simulink library "mblibv1"  (Simulink 6.0)
settings: Solver=ode45  StartTime=0.0  StopTime=10.0  RelTol=1e-3
undefined symbols (not defined in the file or in its folder): gcbh, mech_support
libraries: mblibv1 x10, simulink x5
(part 2 of 2)

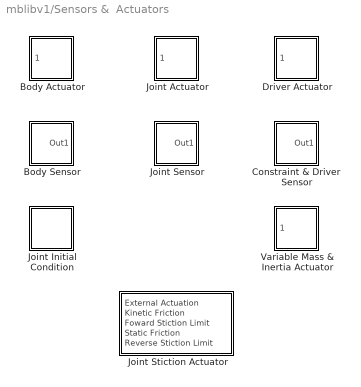
== system mblibv1/Sensors &  Actuators ==
  Body Actuator : Subsystem  LoadFcn=mech_support('LoadFcn',gcbh);  StartFcn=mech_support('StartFcn',gcbh);  StopFcn=mech_support('StopFcn',gcbh);  Opaque=on  mask(msb){PhysicalDomain=Mechanical, PortType=blob, ActuationStyle=Force, AngleUnits=deg, ArcVelocityUnits=deg/s, ArcAccelerationUnits=deg/s^2, CoordPositionUnits=m, VelocityUnits=m/s, AccelerationUnits=m/s^2, ForceUnits=N, TorqueUnits=N-m, ActiveIO=off, Width=1, ClassName=BodyActuatorForceTorque, DialogClass=MechanicalActuatorBlock, ReferenceFrame=Absolute (INERTIAL), Angle=off, CoordPosition=on, Force=on, Torque=off}
      mask help: Actuates a Body with generalized force/torque signal. Vector components specified with respect to reference coordinate system. Input is a Simulink signal. For Body motion or initial condition actuation, press Help.
      mask init:
      | mech_initIO(gcbh);
      settings: CopyFcn=mech_support('CopyFcn',gcbh);  DeleteFcn=mech_support('deleteFcn',gcbh);  UndoDeleteFcn=mech_support('undoDeleteFcn',gcbh);  ModelCloseFcn=mech_support('modelCloseFcn',gcbh);  NameChangeFcn=mech_support('nameChangeFcn',gcbh);  OpenFcn=mech_support('openFcn',gcbh);  CloseFcn=mech_support('CloseFcn',gcbh);
      mask Help: web(mech_help('bodyactuator'))
      mask Display: image(mech_getIcon('b_act.bmp', 'Mechanical'),'center');
  Body Sensor : Subsystem  LoadFcn=mech_support('LoadFcn',gcbh);  StartFcn=mech_support('StartFcn',gcbh);  StopFcn=mech_support('StopFcn',gcbh);  Opaque=on  mask(msb){PhysicalDomain=Mechanical, PortType=blob, Muxed=on, Pose=off, Angle=on, AngleUnits=deg, ArcVelocity=off, ArcVelocityUnits=deg/s, ArcAcceleration=off, ArcAccelerationUnits=deg/s^2, CoordPosition=on, CoordPositionUnits=m, Velocity=off, VelocityUnits=m/s, Acceleration=off, AccelerationUnits=m/s^2, Quaternion=on, QuaternionDT=off, QuaternionDDT=off, QuaternionUnits=off, OutputVector=[1], ActiveIO=off, Width=1, ClassName=BodySensor, DialogClass=MechanicalSensorBlock, ReferenceFrame=Absolute (INERTIAL)}
      mask help: Measures linear/angular position, velocity, and/or acceleration of a Body with respect to a specified coordinate system. Optional rotation matrix for Body orientation. Output is Simulink signal. Multiple output signals can be bundled into one signal.
      mask init:
      | mech_initIO(gcbh);mech_construct(gcbh);
      settings: CopyFcn=mech_support('CopyFcn',gcbh);  DeleteFcn=mech_support('deleteFcn',gcbh);  UndoDeleteFcn=mech_support('undoDeleteFcn',gcbh);  ModelCloseFcn=mech_support('modelCloseFcn',gcbh);  NameChangeFcn=mech_support('nameChangeFcn',gcbh);  OpenFcn=mech_support('openFcn',gcbh);  CloseFcn=mech_support('CloseFcn',gcbh);
      mask Help: web(mech_help('bodysensor'))
      mask Display: image(mech_getIcon('b_sensor.bmp', 'Mechanical'),'center');
  Constraint & Driver  Sensor : Subsystem  LoadFcn=mech_support('LoadFcn',gcbh);  StartFcn=mech_support('StartFcn',gcbh);  StopFcn=mech_support('StopFcn',gcbh);  Opaque=on  mask(msb){PhysicalDomain=Mechanical, ClassName=ConstraintSensor, DialogClass=ConstraintSensorBlock, SensedSide=Base, ReferenceFrame=Absolute (World), ReactionForce=on, ForceUnits=N, ReactionMoment=on, MomentUnits=N-m, Muxed=on, OutputVector=[3 3], ActiveIO=off, Width=1}
      mask help: Measures Constraint/Driver reaction forces/torques between the base (B) and follower (F) Bodies with respect to the selected coordinate system. Outputs are Simulink signals. Force and torque vectors can be bundled into one signal.
      mask init:
      | mech_initIO(gcbh);mech_construct(gcbh);
      settings: CopyFcn=mech_support('CopyFcn',gcbh);  DeleteFcn=mech_support('deleteFcn',gcbh);  UndoDeleteFcn=mech_support('undoDeleteFcn',gcbh);  ModelCloseFcn=mech_support('modelCloseFcn',gcbh);  NameChangeFcn=mech_support('nameChangeFcn',gcbh);  OpenFcn=mech_support('openFcn',gcbh);  CloseFcn=mech_support('CloseFcn',gcbh);
      mask Help: web(mech_help('constraintdriversensor'))
      mask Display: image(mech_getIcon('constr_sen.bmp', 'Mechanical'),'center');
  Driver Actuator : Subsystem  LoadFcn=mech_support('LoadFcn',gcbh);  StartFcn=mech_support('StartFcn',gcbh);  StopFcn=mech_support('StopFcn',gcbh);  Opaque=on  mask(msb){PhysicalDomain=Mechanical, ClassName=ConstraintActuator, DialogClass=ConstraintActuatorBlock, PortType=blob, AngleUnits=deg, ArcVelocityUnits=deg/s, ArcAccelerationUnits=deg/s^2, CoordPositionUnits=m, VelocityUnits=m/s, AccelerationUnits=m/s^2, ActiveIO=off, Width=1}
      mask help: Inputs position, velocity, and acceleration Simulink signals to Driver to drive relative motion between the base (B) and follower (F) Bodies. Base-follower sequence and joint axis determine sign of forward motion. Input signals must be bundled into one signal.
      mask init:
      | mech_initIO(gcbh);
      settings: CopyFcn=mech_support('CopyFcn',gcbh);  DeleteFcn=mech_support('deleteFcn',gcbh);  UndoDeleteFcn=mech_support('undoDeleteFcn',gcbh);  ModelCloseFcn=mech_support('modelCloseFcn',gcbh);  NameChangeFcn=mech_support('nameChangeFcn',gcbh);  OpenFcn=mech_support('openFcn',gcbh);  CloseFcn=mech_support('CloseFcn',gcbh);
      mask Help: web(mech_help('driveractuator'))
      mask Display: image(mech_getIcon('driv_act.bmp', 'Mechanical'),'center');
  Joint Actuator : Subsystem  LoadFcn=mech_support('LoadFcn',gcbh);  StartFcn=mech_support('StartFcn',gcbh);  StopFcn=mech_support('StopFcn',gcbh);  Opaque=on  mask(msb){PhysicalDomain=Mechanical, PortType=blob, ActuationStyle=Force, AngleUnits=deg, ArcVelocityUnits=deg/s, ArcAccelerationUnits=deg/s^2, CoordPositionUnits=m, VelocityUnits=m/s, AccelerationUnits=m/s^2, ForceUnits=N, TorqueUnits=N-m, ActiveIO=off, Width=1, ClassName=JointActuator, DialogClass=MechanicalActuatorBlock, Primitive=None, ReferenceFrame=Absolute (INERTIAL)}
      mask help: Actuates a Joint primitive with generalized force/torque or linear/angular position, velocity, and acceleration motion signals. Base-follower sequence and joint axis determines sign of forward motion. Inputs are Simulink signals. Motion input signals must be bundled into one signal. Connect to Joint block to see Connected to primitive list.
      mask init:
      | mech_initIO(gcbh);
      settings: CopyFcn=mech_support('CopyFcn',gcbh);  DeleteFcn=mech_support('deleteFcn',gcbh);  UndoDeleteFcn=mech_support('undoDeleteFcn',gcbh);  ModelCloseFcn=mech_support('modelCloseFcn',gcbh);  NameChangeFcn=mech_support('nameChangeFcn',gcbh);  OpenFcn=mech_support('openFcn',gcbh);  CloseFcn=mech_support('CloseFcn',gcbh);
      mask Help: web(mech_help('jointactuator'))
      mask Display: image(mech_getIcon('j_act.bmp', 'Mechanical'),'center');
  Joint Initial Condition : Subsystem  LoadFcn=mech_support('LoadFcn',gcbh);  StartFcn=mech_support('StartFcn',gcbh);  StopFcn=mech_support('StopFcn',gcbh);  Opaque=on  mask(msb){PhysicalDomain=Mechanical, ClassName=InitialCondition, DialogClass=InitialConditionBlock, Primitive=, CoordPosition=, Velocity=, AngleUnits=, ArcVelocityUnits=, CoordPositionUnits=, VelocityUnits=, InitialConditions=P1$false$0$m$rad$0$m/s$rad/s#P2$false$0$m$rad$0$m/s$rad/s#P3$false$0$m$rad$0$m/s$rad/s#R1$false$0$m$rad$0$m/s$rad/s#R2$false$0$m$rad$0$m/s$rad/s#R3$false$0$m$rad$0$m/s$rad/s#S$false$0$m$rad$0$m/s$rad/s}
      mask help: Sets the initial linear/angular position and velocity of some or all of the primitives in a Joint. Connect to a Joint to see a list of its primitives.
      settings: CopyFcn=mech_support('CopyFcn',gcbh);  DeleteFcn=mech_support('deleteFcn',gcbh);  UndoDeleteFcn=mech_support('undoDeleteFcn',gcbh);  ModelCloseFcn=mech_support('modelCloseFcn',gcbh);  PreSaveFcn=mech_support('PreSaveFcn');  PostSaveFcn=mech_support('PostSaveFcn');  NameChangeFcn=mech_support('nameChangeFcn',gcbh);  OpenFcn=mech_support('openFcn',gcbh);  CloseFcn=mech_support('CloseFcn',gcbh);
      mask Help: web(mech_help('jointinitialconditionactuator'))
      mask Display: image(mech_getIcon('init_cond.bmp', 'Mechanical'),'center');
  Joint Sensor : Subsystem  LoadFcn=mech_support('LoadFcn',gcbh);  StartFcn=mech_support('StartFcn',gcbh);  StopFcn=mech_support('StopFcn',gcbh);  Opaque=on  mask(msb){PhysicalDomain=Mechanical, PortType=blob, Muxed=on, Pose=off, Angle=on, AngleUnits=deg, ArcVelocity=off, ArcVelocityUnits=deg/s, ArcAcceleration=off, ArcAccelerationUnits=deg/s^2, CoordPosition=on, CoordPositionUnits=m, Velocity=off, VelocityUnits=m/s, Acceleration=off, AccelerationUnits=m/s^2, Quaternion=on, QuaternionDT=off, QuaternionDDT=off, QuaternionUnits=off, OutputVector=[1], ActiveIO=off, Width=1, ClassName=JointSensor, DialogClass=MechanicalSensorBlock, Primitive=None, Force=off, ForceUnits=N, Torque=off, TorqueUnits=N-m, ReferenceFrame=Absolute (INERTIAL), ReactionSensedSide=Base, ReactionReferenceFrame=Absolute (World), ReactionForce=off, ReactionForceUnits=N, ReactionMoment=off, ReactionMomentUnits=N-m}
      mask help: Measures linear/angular position, velocity, acceleration, computed force/torque and/or reaction force/torque of a Joint primitive. Spherical measured by quaternion. Base-follower sequence and joint axis determine sign of forward motion. Outputs are Simulink signals. Multiple output signals can be bundled into one signal. Connect to Joint block to see Connected to primitive list.
      mask init:
      | mech_initIO(gcbh);mech_construct(gcbh);
      settings: CopyFcn=mech_support('CopyFcn',gcbh);  DeleteFcn=mech_support('deleteFcn',gcbh);  UndoDeleteFcn=mech_support('undoDeleteFcn',gcbh);  ModelCloseFcn=mech_support('modelCloseFcn',gcbh);  NameChangeFcn=mech_support('nameChangeFcn',gcbh);  OpenFcn=mech_support('openFcn',gcbh);  CloseFcn=mech_support('CloseFcn',gcbh);
      mask Help: web(mech_help('jointsensor'))
      mask Display: image(mech_getIcon('j_sensor.bmp', 'Mechanical'),'center');
  Joint Stiction Actuator : Subsystem  LoadFcn=mech_support('LoadFcn',gcbh);  StartFcn=mech_support('StartFcn',gcbh);  StopFcn=mech_support('StopFcn',gcbh);  Opaque=on  mask(msb){PhysicalDomain=Mechanical, PortType=blob, ActuationStyle=Force, AngleUnits=deg, ArcVelocityUnits=deg/s, ArcAccelerationUnits=deg/s^2, CoordPositionUnits=m, VelocityUnits=m/s, AccelerationUnits=m/s^2, ForceUnits=N, TorqueUnits=N-m, ActiveIO=off, Width=1, ClassName=JointStictionActuator, DialogClass=EventActuatorBlock, Primitive=None, FrictionalForceUnits=N, ExternalForceUnits=N, FrictionalTorqueUnits=N-m, ExternalTorqueUnits=N-m, LockingTolerance=1e-2}
      mask help: Actuates a Joint primitive with stiction force/torque. Locked if static friction remains within range of forward and reverse stiction limits. External actuation and kinetic friction require units. Velocity threshold in MKS (SI) units. Base-follower sequence and joint axis determine sign of forward motion. Inputs are Simulink signals. Connect to Joint block to see the Connected to primitive list.
      mask init:
      | mech_initIO(gcbh);
      settings: CopyFcn=mech_support('CopyFcn',gcbh);  DeleteFcn=mech_support('deleteFcn',gcbh);  UndoDeleteFcn=mech_support('undoDeleteFcn',gcbh);  ModelCloseFcn=mech_support('modelCloseFcn',gcbh);  NameChangeFcn=mech_support('nameChangeFcn',gcbh);  OpenFcn=mech_support('openFcn',gcbh);  CloseFcn=mech_support('CloseFcn',gcbh);
      mask Help: web(mech_help('jointstictionactuator'))
  Variable Mass & Inertia Actuator : Subsystem  LoadFcn=mech_support('LoadFcn',gcbh);  StartFcn=mech_support('StartFcn',gcbh);  StopFcn=mech_support('StopFcn',gcbh);  Opaque=on  mask(msb){PhysicalDomain=Mechanical, PortType=blob, ActuationStyle=MassInertia, AngleUnits=deg, ArcVelocityUnits=deg/s, ArcAccelerationUnits=deg/s^2, CoordPositionUnits=m, VelocityUnits=m/s, AccelerationUnits=m/s^2, ForceUnits=N, TorqueUnits=N-m, ActiveIO=off, Width=1, ClassName=BodyActuatorMassInertia, DialogClass=VariableMassInertiaActuatorBlock, Mass=on, Inertia=off, ReferenceFrame=Local (body CS), MassUnits=kg, InertiaUnits=kg*m^2}
      mask help: Varies the mass and/or inertia tensor of the connected Body. Attaches to the connected Body coordinate system (CS) an invisible body of time-varying mass and/or inertia tensor. Time-varying mass and inertia tensor are transformed from the attached CS to the new common center of gravity and added to the values supplied in the Body dialog. Multiple time-varying masses and inertia tensors can be added to a Body. Input is a Simulink signal with one, nine, or ten components.
      mask init:
      | mech_initIO(gcbh);
      settings: CopyFcn=mech_support('CopyFcn',gcbh);  DeleteFcn=mech_support('deleteFcn',gcbh);  UndoDeleteFcn=mech_support('undoDeleteFcn',gcbh);  ModelCloseFcn=mech_support('modelCloseFcn',gcbh);  NameChangeFcn=mech_support('nameChangeFcn',gcbh);  OpenFcn=mech_support('openFcn',gcbh);  CloseFcn=mech_support('CloseFcn',gcbh);
      mask Help: web(mech_help('variablemassinertiaactuator'))
      mask Display: image(mech_getIcon('vmi_act.bmp', 'Mechanical'),'center');

== system mblibv1/Utilities ==
  Continuous Angle : Subsystem  Tag=Factory continuousAngle  AncestorBlock=plantlib/Smooth Angle  mask{rad=deg, rads=deg/s}
      mask prompts: rad "Angle measured in:"; rads "Rate measured in:"
      mask help: Outputs a continuous, unbounded angle given a discontinuous, bounded angle and the angular velocity. Choose units for the angle and the angular velocity (rate).
      mask Help: web(mech_help('continuousangle'))
      mask StyleString: popup(rad|deg),popup(rad/s|deg/s)
  Convert from Rotation Matrix to Virtual Reality Toolbox : S-Function  Tag=Pose2VR  FunctionName=sfun_pose2vr
      mask Type: RotationMatrix2VR
      mask Description: Transforms body orientation representations. Converts a 3 x 3 rotation matrix to a 4-component vector, a spatial unit vector plus a rotation angle about that vector. The input must be a 9-element vector representing the rotation matrix column-wise. The output format is that required by the Virtual Reality Toolbox for specifying orientation.
      mask Help: web(mech_help('rotationmatrix2vr'))
      mask Display: disp('RotationMatrix2VR')
  Mechanical Branching Bar : PMComponent  LoadFcn=mech_support('LoadFcn',gcbh);  StartFcn=mech_support('StartFcn',gcbh);  StopFcn=mech_support('StopFcn',gcbh);  PhysicalDomain=mechanical  SubClassName=Unknown  LeftPortType=blob  RightPortType=blob  LConnTagsString=_newl0  RConnTagsString=SA0|SA1  mask(msb){ClassName=BranchingBar, DialogClass=MechanicalBranchingBarBlock, NumSAPorts=2}
      mask help: Maps multiple sensor/actuator lines to one sensor/actuator port. On a Body, connects many sensor/actuator lines to one Body coordinate system. On a Joint, Constraint, or Driver, connects many sensor/actuator lines to one sensor/actuator port. Allows choice of primitives on Joints, reactions forces/torques on Constraints and Drivers, and motion actuation on Drivers.
      settings: CopyFcn=mech_support('CopyFcn',gcbh);  DeleteFcn=mech_support('deleteFcn',gcbh);  UndoDeleteFcn=mech_support('undoDeleteFcn',gcbh);  ModelCloseFcn=mech_support('modelCloseFcn',gcbh);  NameChangeFcn=mech_support('nameChangeFcn',gcbh);  OpenFcn=mech_support('openFcn',gcbh);  CloseFcn=mech_support('CloseFcn',gcbh);
      mask Help: web(mech_help('mechanicalbranchingbar'))
      mask Display: image(mech_getIcon('branchingbar.bmp', 'Mechanical'));
  Connection Port : PMIOPort  Tag=PMCPort  Port=1  Side=Left

== system mblibv1/Bodies/Ground ==
  out : PMIOPort  Port=1  Side=Right

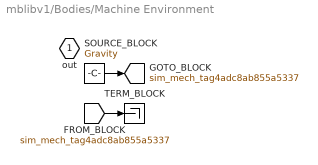
== system mblibv1/Bodies/Machine Environment ==
  SOURCE_BLOCK : Constant  Value=Gravity
  TERM_BLOCK : Terminator
  out : PMIOPort  Port=1  Side=Right
  tag scope: sim_mech_tag4adc8ab855a5337=global
  wires:
  SOURCE_BLOCK/1 -> [sim_mech_tag4adc8ab855a5337]
  [sim_mech_tag4adc8ab855a5337] -> TERM_BLOCK/1

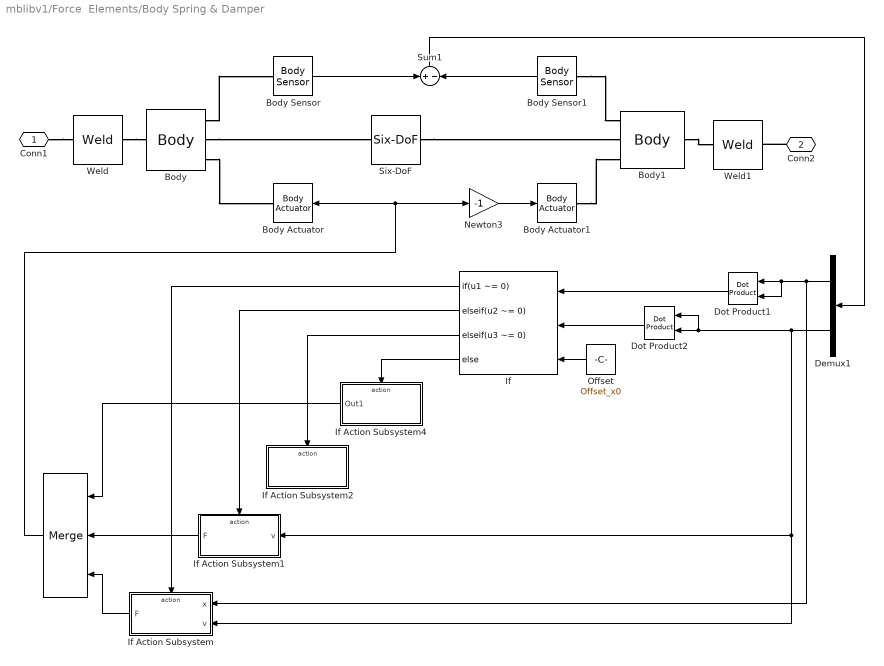
== system mblibv1/Force  Elements/Body Spring & Damper ==
  " " : Merge  Orientation=left  Inputs=3
  Body : mblibv1/Bodies/Body  PhysicalDomain=mechanical  SubClassName=Unknown  LeftPortType=workingframe  RightPortType=workingframe  LConnTagsString=CS1  RConnTagsString=CS2|CS3|CS4  DialogClass=MechanicalBodyBlock  Mass=0  MassUnits=kg  InertiaUnits=kg*m^2  Inertia=zeros(3, 3)  Shape=Cylinder  ShapeDims=[1 1]  ShapeUnits=m  ShapeUse=false  Density=1  DensityUnits=kg/m^3  DensityUse=false  CG=Left$CG$[0 0 0]$CS1$CS1$m$[0 0 0]$Euler X-Y-Z$deg$WORLD$false  WorkingFrames=Left$CS1$[0 0 0]$ADJOINING$ADJOINING$m$[0 0 0]$Euler X-Y-Z$deg$WORLD$true#Right$CS2$[0 0 0]$CS1$CS1$m$[0 0 0]$Euler X-Y-Z$deg$WORLD$true#Right$CS3$[0 0 0]$CS1$CS1$m$[0 0 0]$Euler X-Y-Z$deg$WORLD$true#Right$CS4$[0 0 0]$CS1$CS1$m$[0 0 0]$Euler X-Y-Z$deg$WORLD$true
  Body Actuator : mblibv1/Sensors &  Actuators/Body Actuator  Orientation=left  Opaque=on  PhysicalDomain=Mechanical  PortType=blob  ActuationStyle=Force  AngleUnits=deg  ArcVelocityUnits=deg/s  ArcAccelerationUnits=deg/s^2  CoordPositionUnits=m  VelocityUnits=m/s  AccelerationUnits=m/s^2  ForceUnits=N  TorqueUnits=N-m  ActiveIO=off  Width=3  DialogClass=MechanicalActuatorBlock  ReferenceFrame=Absolute (INERTIAL)  Angle=off  CoordPosition=on  Force=on  Torque=off
  Body Actuator1 : mblibv1/Sensors &  Actuators/Body Actuator  Opaque=on  PhysicalDomain=Mechanical  PortType=blob  ActuationStyle=Force  AngleUnits=deg  ArcVelocityUnits=deg/s  ArcAccelerationUnits=deg/s^2  CoordPositionUnits=m  VelocityUnits=m/s  AccelerationUnits=m/s^2  ForceUnits=N  TorqueUnits=N-m  ActiveIO=off  Width=3  DialogClass=MechanicalActuatorBlock  ReferenceFrame=Absolute (INERTIAL)  Angle=off  CoordPosition=on  Force=on  Torque=off
  Body Sensor : mblibv1/Sensors &  Actuators/Body Sensor  Opaque=on  PhysicalDomain=Mechanical  PortType=blob  Muxed=on  Pose=off  Angle=on  AngleUnits=deg  ArcVelocity=off  ArcVelocityUnits=deg/s  ArcAcceleration=off  ArcAccelerationUnits=deg/s^2  CoordPosition=on  CoordPositionUnits=m  Velocity=on  VelocityUnits=m/s  Acceleration=off  AccelerationUnits=m/s^2  Quaternion=on  QuaternionDT=off  QuaternionDDT=off  QuaternionUnits=deg  OutputVector=[ 3 3 ]  ActiveIO=off  Width=6  DialogClass=MechanicalSensorBlock  ReferenceFrame=Absolute (World)
  Body Sensor1 : mblibv1/Sensors &  Actuators/Body Sensor  Orientation=left  Opaque=on  PhysicalDomain=Mechanical  PortType=blob  Muxed=on  Pose=off  Angle=on  AngleUnits=deg  ArcVelocity=off  ArcVelocityUnits=deg/s  ArcAcceleration=off  ArcAccelerationUnits=deg/s^2  CoordPosition=on  CoordPositionUnits=m  Velocity=on  VelocityUnits=m/s  Acceleration=off  AccelerationUnits=m/s^2  Quaternion=on  QuaternionDT=off  QuaternionDDT=off  QuaternionUnits=deg  OutputVector=[ 3 3 ]  ActiveIO=off  Width=6  DialogClass=MechanicalSensorBlock  ReferenceFrame=Absolute (World)
  Body1 : mblibv1/Bodies/Body  PhysicalDomain=mechanical  SubClassName=Unknown  LeftPortType=workingframe  RightPortType=workingframe  LConnTagsString=CS1|CS3|CS4  RConnTagsString=CS2  DialogClass=MechanicalBodyBlock  Mass=0  MassUnits=kg  InertiaUnits=kg*m^2  Inertia=zeros(3, 3)  Shape=Cylinder  ShapeDims=[1 1]  ShapeUnits=m  ShapeUse=false  Density=1  DensityUnits=kg/m^3  DensityUse=false  CG=Left$CG$[0 0 0]$CS2$CS2$m$[0 0 0]$Euler X-Y-Z$deg$WORLD$false  WorkingFrames=Left$CS1$[0 0 0]$CS2$CS2$m$[0 0 0]$Euler X-Y-Z$deg$WORLD$true#Right$CS2$[0 0 0]$ADJOINING$ADJOINING$m$[0 0 0]$Euler X-Y-Z$deg$WORLD$true#Left$CS3$[0 0 0]$CS2$CS2$m$[0 0 0]$Euler X-Y-Z$deg$WORLD$true#Left$CS4$[0 0 0]$CS2$CS2$m$[0 0 0]$Euler X-Y-Z$deg$WORLD$true
  Demux1 : Demux  Orientation=left  Outputs=2
  Dot Product1 : simulink/Math Operations/Dot Product  Orientation=left  OutDataType=sfix(16)  OutScaling=2^-10  DoSatur=off
  Dot Product2 : simulink/Math Operations/Dot Product  Orientation=left  OutDataType=sfix(16)  OutScaling=2^-10  DoSatur=off
  If : If  Orientation=left  NumInputs=3  IfExpression=u1 ~= 0  ElseIfExpressions=u2 ~= 0, u3 ~= 0  ZeroCross=off
  If Action Subsystem : Subsystem  Orientation=left  TreatAsAtomicUnit=on
  If Action Subsystem1 : Subsystem  Orientation=left  TreatAsAtomicUnit=on
  If Action Subsystem2 : Subsystem  Orientation=left  TreatAsAtomicUnit=on
  If Action Subsystem4 : Subsystem  Orientation=left  TreatAsAtomicUnit=on
  Newton3 : Gain  Gain=-1  SaturateOnIntegerOverflow=on
  Offset : Constant  Orientation=left  Value=Offset_x0  VectorParams1D=off
  Six-DoF : mblibv1/Joints/Six-DoF  PhysicalDomain=mechanical  SubClassName=Unknown  LeftPortType=blob  RightPortType=blob  LConnTagsString=__newl0  RConnTagsString=__newr0  NumSAPorts=0  CutJoint=on  MarkAsCut=off  Primitives=prismatic_prismatic_prismatic_spherical  PrimitiveProps=P1$WORLD$[1 0 0]$prismatic#P2$WORLD$[0 1 0]$prismatic#P3$WORLD$[0 0 1]$prismatic#S$WORLD$[0 0 0]$spherical  DialogClass=JointBlock
  Sum1 : Sum  Orientation=up  Inputs=+-  SaturateOnIntegerOverflow=on
  Weld : mblibv1/Joints/Weld  PhysicalDomain=mechanical  SubClassName=Unknown  LeftPortType=blob  RightPortType=blob  LConnTagsString=__newl0  RConnTagsString=__newr0  NumSAPorts=0  CutJoint=off  MarkAsCut=off  Primitives=weld  PrimitiveProps=W$INERTIAL$[0 0 0]$weld  DialogClass=JointBlock
  Weld1 : mblibv1/Joints/Weld  PhysicalDomain=mechanical  SubClassName=Unknown  LeftPortType=blob  RightPortType=blob  LConnTagsString=__newl0  RConnTagsString=__newr0  NumSAPorts=0  CutJoint=off  MarkAsCut=off  Primitives=weld  PrimitiveProps=W$INERTIAL$[0 0 0]$weld  DialogClass=JointBlock
  Conn1 : PMIOPort  Port=1  Side=Left
  Conn2 : PMIOPort  Orientation=left  Port=2  Side=Right
  wires:
  Newton3/1 -> Body Actuator1/1
  Sum1/1 -> Demux1/1
  Body Sensor1/1 -> Sum1/2
  Body Sensor/1 -> Sum1/1
  If/1 -> If Action Subsystem/Action
  If/2 -> If Action Subsystem1/Action
  If/3 -> If Action Subsystem2/Action
  If/4 -> If Action Subsystem4/Action
  If Action Subsystem1/1(F) -> " "/2
  If Action Subsystem/1(F) -> " "/3
  If Action Subsystem4/1(Out1) -> " "/1
  " "/1 -> Newton3/1, Body Actuator/1
  Dot Product1/1 -> If/1
  Offset/1 -> If/3
  Demux1/1 -> If Action Subsystem/1(x), Dot Product1/1, Dot Product1/2
  Demux1/2 -> If Action Subsystem/2(v), If Action Subsystem1/1(v), Dot Product2/1, Dot Product2/2
  Dot Product2/1 -> If/2
  connections:
  Six-DoF/RConn1 -- Body1/LConn2
  Body/RConn2 -- Six-DoF/LConn1
  Body/RConn3 -- Body Actuator/RConn1
  Body Actuator1/RConn1 -- Body1/LConn3
  Weld/RConn1 -- Body/LConn1
  Body/RConn1 -- Body Sensor/LConn1
  Body Sensor1/LConn1 -- Body1/LConn1
  Body1/RConn1 -- Weld1/LConn1
  Conn1/RConn1 -- Weld/LConn1
  Conn2/RConn1 -- Weld1/RConn1

== system mblibv1/Force  Elements/Joint Spring & Damper ==
  Mechanical Branching Bar : mblibv1/Utilities/Mechanical Branching Bar  PhysicalDomain=mechanical  SubClassName=Unknown  LeftPortType=blob  RightPortType=blob  LConnTagsString=_newl0  RConnTagsString=SA1|SA2|SA3|SA4|SA5|SA6|SA7|SA8|SA9|SA10|SA11|SA12|SA13|SA14  DialogClass=MechanicalBranchingBarBlock  NumSAPorts=14
  Conn1 : PMIOPort  Port=1  Side=Left
  connections:
  Mechanical Branching Bar/LConn1 -- Conn1/RConn1

== system mblibv1/Joints/Disassembled Joints ==
  Disassembled Cylindrical : PMComponent  LoadFcn=mech_support('LoadFcn',gcbh);  StartFcn=mech_support('StartFcn',gcbh);  StopFcn=mech_support('StopFcn',gcbh);  PhysicalDomain=mechanical  SubClassName=disassembled_cylindrical_joint  LeftPortType=blob  RightPortType=blob  LConnTagsString=__newl0  RConnTagsString=__newr0  mask(msb){DialogClass=JointBlock, Primitives=prismatic_prismatic, PrimitiveProps=Base$INERTIAL$[1 0 0]$prismatic#Follower$INERTIAL$[0 1 0]$prismatic, ClassName=DisassembledCylindrical}
      mask help: Creates two misaligned cylindrical joints, one attached to the base (B) and other attached to the follower (F) Body. Axes and Body coordinate systems are automatically aligned at simulation start. Cannot be sensed or actuated. Must only be used in closed loops.
      settings: CopyFcn=mech_support('CopyFcn',gcbh);  DeleteFcn=mech_support('deleteFcn',gcbh);  UndoDeleteFcn=mech_support('undoDeleteFcn',gcbh);  ModelCloseFcn=mech_support('modelCloseFcn',gcbh);  NameChangeFcn=mech_support('nameChangeFcn',gcbh);  OpenFcn=mech_support('openFcn',gcbh);  CloseFcn=mech_support('CloseFcn',gcbh);
      mask Help: web(mech_help('disassembledcylindrical'))
      mask Display: image(mech_getIcon('cylindrical.bmp', 'Mechanical'),'center');image(mech_getIcon('dis_affordance.bmp', 'Mechanical'),'bottom-left');color('magenta');port_label('LConn',1,'B'); port_label('RConn',1,'F')
  Disassembled Prismatic : PMComponent  LoadFcn=mech_support('LoadFcn',gcbh);  StartFcn=mech_support('StartFcn',gcbh);  StopFcn=mech_support('StopFcn',gcbh);  PhysicalDomain=mechanical  SubClassName=disassembled_prismatic_joint  LeftPortType=blob  RightPortType=blob  LConnTagsString=__newl0  RConnTagsString=__newr0  mask(msb){DialogClass=JointBlock, Primitives=prismatic_prismatic, PrimitiveProps=Base$INERTIAL$[1 0 0]$prismatic#Follower$INERTIAL$[0 1 0]$prismatic, ClassName=DisassembledPrismatic}
      mask help: Creates two misaligned primitive prismatic axes, one attached to the base (B) and other attached to the follower (F) Body. Axes and Body coordinate systems are automatically aligned at simulation start. Cannot be sensed or actuated. Must only be used in closed loops.
      settings: CopyFcn=mech_support('CopyFcn',gcbh);  DeleteFcn=mech_support('deleteFcn',gcbh);  UndoDeleteFcn=mech_support('undoDeleteFcn',gcbh);  ModelCloseFcn=mech_support('modelCloseFcn',gcbh);  NameChangeFcn=mech_support('nameChangeFcn',gcbh);  OpenFcn=mech_support('openFcn',gcbh);  CloseFcn=mech_support('CloseFcn',gcbh);
      mask Help: web(mech_help('disassembledprismatic'))
      mask Display: image(mech_getIcon('prismatic.bmp', 'Mechanical'),'center');image(mech_getIcon('dis_affordance.bmp', 'Mechanical'),'bottom-left');color('magenta');port_label('LConn',1,'B'); port_label('RConn',1,'F')
  Disassembled Revolute : PMComponent  LoadFcn=mech_support('LoadFcn',gcbh);  StartFcn=mech_support('StartFcn',gcbh);  StopFcn=mech_support('StopFcn',gcbh);  PhysicalDomain=mechanical  SubClassName=disassembled_revolute_joint  LeftPortType=blob  RightPortType=blob  LConnTagsString=__newl0  RConnTagsString=__newr0  mask(msb){DialogClass=JointBlock, Primitives=prismatic_prismatic, PrimitiveProps=Base$INERTIAL$[1 0 0]$prismatic#Follower$INERTIAL$[0 1 0]$prismatic, ClassName=DisassembledRevolute}
      mask help: Creates two misaligned primitive revolute axes, one attached to the base (B) and other attached to the follower (F) Body. Axes and Body coordinate systems are automatically aligned at simulation start. Cannot be sensed or actuated. Must only be used in closed loops.
      settings: CopyFcn=mech_support('CopyFcn',gcbh);  DeleteFcn=mech_support('deleteFcn',gcbh);  UndoDeleteFcn=mech_support('undoDeleteFcn',gcbh);  ModelCloseFcn=mech_support('modelCloseFcn',gcbh);  NameChangeFcn=mech_support('nameChangeFcn',gcbh);  OpenFcn=mech_support('openFcn',gcbh);  CloseFcn=mech_support('CloseFcn',gcbh);
      mask Help: web(mech_help('disassembledrevolute'))
      mask Display: image(mech_getIcon('revolute.bmp', 'Mechanical'),'center');image(mech_getIcon('dis_affordance.bmp', 'Mechanical'),'bottom-left');color('magenta');port_label('LConn',1,'B'); port_label('RConn',1,'F')
  Disassembled Spherical : PMComponent  LoadFcn=mech_support('LoadFcn',gcbh);  StartFcn=mech_support('StartFcn',gcbh);  StopFcn=mech_support('StopFcn',gcbh);  PhysicalDomain=mechanical  SubClassName=disassembled_spherical_joint  LeftPortType=blob  RightPortType=blob  LConnTagsString=__newl0  RConnTagsString=__newr0  mask(msb){DialogClass=JointBlock, Primitives=prismatic_prismatic, PrimitiveProps=Base$INERTIAL$[1 0 0]$prismatic#Follower$INERTIAL$[0 1 0]$prismatic, ClassName=DisassembledSpherical}
      mask help: Creates two spatially dislocated origins of the base (B) and the follower (F) Body coordinate systems as spherical pivots attached to each Body. The origins/pivots are automatically collocated at simulation start. Cannot be sensed or actuated. Must only be used in closed loops.
      settings: CopyFcn=mech_support('CopyFcn',gcbh);  DeleteFcn=mech_support('deleteFcn',gcbh);  UndoDeleteFcn=mech_support('undoDeleteFcn',gcbh);  ModelCloseFcn=mech_support('modelCloseFcn',gcbh);  NameChangeFcn=mech_support('nameChangeFcn',gcbh);  OpenFcn=mech_support('openFcn',gcbh);  CloseFcn=mech_support('CloseFcn',gcbh);
      mask Help: web(mech_help('disassembledspherical'))
      mask Display: image(mech_getIcon('sphere.bmp', 'Mechanical'),'center');image(mech_getIcon('dis_affordance.bmp', 'Mechanical'),'bottom-left');color('magenta');port_label('LConn',1,'B'); port_label('RConn',1,'F')

== system mblibv1/Joints/Massless Connectors ==
  Revolute-Revolute : PMComponent  LoadFcn=mech_support('LoadFcn',gcbh);  StartFcn=mech_support('StartFcn',gcbh);  StopFcn=mech_support('StopFcn',gcbh);  PhysicalDomain=mechanical  SubClassName=massless_connector  LeftPortType=blob  RightPortType=blob  LConnTagsString=__newl0  RConnTagsString=__newr0  mask(msb){NumSAPorts=0, CutJoint=off, MarkAsCut=off, Primitives=revolute_revolute, PrimitiveProps=R1$INERTIAL$[0 0 1]$revolute#R2$INERTIAL$[0 1 0]$revolute, ClassName=MasslessRR, DialogClass=JointBlock}
      mask help: Creates two separated revolute axes on the base (B) and follower (F) Bodies. The separation vector between the base and follower Body coordinate systems changes, but the separation distance is constant. This joint becomes singular if the two revolute axes align with the separation vector. Cannot be sensed or actuated.
      settings: CopyFcn=mech_support('CopyFcn',gcbh);  DeleteFcn=mech_support('deleteFcn',gcbh);  UndoDeleteFcn=mech_support('undoDeleteFcn',gcbh);  ModelCloseFcn=mech_support('modelCloseFcn',gcbh);  PreSaveFcn=mech_support('PreSaveFcn');  PostSaveFcn=mech_support('PostSaveFcn');  NameChangeFcn=mech_support('nameChangeFcn',gcbh);  OpenFcn=mech_support('openFcn',gcbh);  CloseFcn=mech_support('CloseFcn',gcbh);
      mask Help: web(mech_help('revoluterevolute'))
      mask Display: image(mech_getIcon('rr_cplr.bmp', 'Mechanical'),'center');color('red');text(mech_cutAffordance('offset', gcbh) - 2, 0, mech_cutAffordance('text', gcbh),'HorizontalAlignment', 'right','VerticalAlignment', 'bottom');color('magenta');port_label('LConn', 1, 'B');port_label('RConn', 1, 'F');
  Revolute-Spherical : PMComponent  LoadFcn=mech_support('LoadFcn',gcbh);  StartFcn=mech_support('StartFcn',gcbh);  StopFcn=mech_support('StopFcn',gcbh);  PhysicalDomain=mechanical  SubClassName=massless_connector  LeftPortType=blob  RightPortType=blob  LConnTagsString=__newl0  RConnTagsString=__newr0  mask(msb){NumSAPorts=0, CutJoint=off, MarkAsCut=off, Primitives=revolute_spherical, PrimitiveProps=R1$INERTIAL$[0 0 1]$revolute#S$INERTIAL$[0 0 0]$spherical, ClassName=MasslessRS, DialogClass=JointBlock}
      mask help: Creates separated revolute axis on the base (B) and spherical pivot point on the follower (F) Bodies. The separation vector between the base and follower Body coordinate systems changes, but the separation distance is constant. This joint becomes singular if the revolute axis aligns with the separation vector. Cannot be sensed or actuated.
      settings: CopyFcn=mech_support('CopyFcn',gcbh);  DeleteFcn=mech_support('deleteFcn',gcbh);  UndoDeleteFcn=mech_support('undoDeleteFcn',gcbh);  ModelCloseFcn=mech_support('modelCloseFcn',gcbh);  PreSaveFcn=mech_support('PreSaveFcn');  PostSaveFcn=mech_support('PostSaveFcn');  NameChangeFcn=mech_support('nameChangeFcn',gcbh);  OpenFcn=mech_support('openFcn',gcbh);  CloseFcn=mech_support('CloseFcn',gcbh);
      mask Help: web(mech_help('revolutespherical'))
      mask Display: image(mech_getIcon('rs_cplr.bmp', 'Mechanical'),'center');color('red');text(mech_cutAffordance('offset', gcbh) - 2, 0, mech_cutAffordance('text', gcbh),'HorizontalAlignment', 'right','VerticalAlignment', 'bottom');color('magenta');port_label('LConn', 1, 'B');port_label('RConn', 1, 'F');
  Spherical-Spherical : PMComponent  LoadFcn=mech_support('LoadFcn',gcbh);  StartFcn=mech_support('StartFcn',gcbh);  StopFcn=mech_support('StopFcn',gcbh);  PhysicalDomain=mechanical  SubClassName=massless_connector  LeftPortType=blob  RightPortType=blob  LConnTagsString=__newl0  RConnTagsString=__newr0  mask(msb){NumSAPorts=0, CutJoint=off, MarkAsCut=off, Primitives=spherical_spherical, PrimitiveProps=S1$INERTIAL$[0 0 0]$spherical#S2$INERTIAL$[0 0 0]$spherical, ClassName=MasslessSS, DialogClass=JointBlock}
      mask help: Creates two separated spherical pivot points on the base (B) and follower (F) Bodies. The separation vector between the base and follower Body coordinate systems changes, but the separation distance is constant. Cannot be sensed or actuated.
      settings: CopyFcn=mech_support('CopyFcn',gcbh);  DeleteFcn=mech_support('deleteFcn',gcbh);  UndoDeleteFcn=mech_support('undoDeleteFcn',gcbh);  ModelCloseFcn=mech_support('modelCloseFcn',gcbh);  PreSaveFcn=mech_support('PreSaveFcn');  PostSaveFcn=mech_support('PostSaveFcn');  NameChangeFcn=mech_support('nameChangeFcn',gcbh);  OpenFcn=mech_support('openFcn',gcbh);  CloseFcn=mech_support('CloseFcn',gcbh);
      mask Help: web(mech_help('sphericalspherical'))
      mask Display: image(mech_getIcon('ss_cplr.bmp', 'Mechanical'),'center');color('red');text(mech_cutAffordance('offset', gcbh) - 2, 0, mech_cutAffordance('text', gcbh),'HorizontalAlignment', 'right','VerticalAlignment', 'bottom');color('magenta');port_label('LConn', 1, 'B');port_label('RConn', 1, 'F');

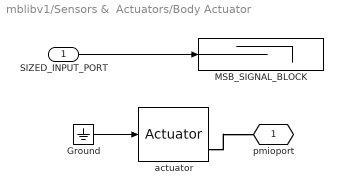
== system mblibv1/Sensors &  Actuators/Body Actuator ==
  SIZED_INPUT_PORT : Inport  Port=1  PortDimensions=1  LatchInput=off
  Ground : Ground
  MSB_SIGNAL_BLOCK : Terminator
  actuator : Actuator  PhysicalDomain=generic  SubClassName=Unknown  PortType=Generic
  pmioport : PMIOPort  Orientation=left  Port=1  Side=Right
  wires:
  SIZED_INPUT_PORT/1 -> MSB_SIGNAL_BLOCK/1
  Ground/1 -> actuator/1
  connections:
  actuator/RConn1 -- pmioport/RConn1

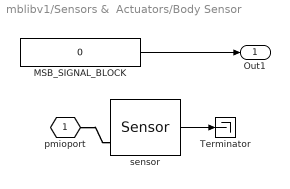
== system mblibv1/Sensors &  Actuators/Body Sensor ==
  MSB_SIGNAL_BLOCK : Constant  Value=0
  Terminator : Terminator
  sensor : Sensor  Tag=Factory sensor  PhysicalDomain=generic  SubClassName=Unknown  PortType=Generic
  pmioport : PMIOPort  Port=1  Side=Left
  Out1 : Outport
  wires:
  sensor/1 -> Terminator/1
  MSB_SIGNAL_BLOCK/1 -> Out1/1
  connections:
  pmioport/RConn1 -- sensor/LConn1

== system mblibv1/Sensors &  Actuators/Constraint & Driver  Sensor ==
  MSB_SIGNAL_BLOCK : Constant  Value=0
  Terminator : Terminator
  sensor : Sensor  Tag=Factory sensor  PhysicalDomain=generic  SubClassName=Unknown  PortType=Generic
  pmioport : PMIOPort  Port=1  Side=Left
  Out1 : Outport
  wires:
  sensor/1 -> Terminator/1
  MSB_SIGNAL_BLOCK/1 -> Out1/1
  connections:
  pmioport/RConn1 -- sensor/LConn1

== system mblibv1/Sensors &  Actuators/Driver Actuator ==
  SIZED_INPUT_PORT : Inport  Port=1  PortDimensions=1  LatchInput=off
  Ground : Ground
  MSB_SIGNAL_BLOCK : Terminator
  actuator : Actuator  PhysicalDomain=generic  SubClassName=Unknown  PortType=Generic
  pmioport : PMIOPort  Orientation=left  Port=1  Side=Right
  wires:
  SIZED_INPUT_PORT/1 -> MSB_SIGNAL_BLOCK/1
  Ground/1 -> actuator/1
  connections:
  actuator/RConn1 -- pmioport/RConn1

== system mblibv1/Sensors &  Actuators/Joint Actuator ==
  SIZED_INPUT_PORT : Inport  Port=1  PortDimensions=1  LatchInput=off
  Ground : Ground
  MSB_SIGNAL_BLOCK : Terminator
  actuator : Actuator  PhysicalDomain=generic  SubClassName=Unknown  PortType=Generic
  pmioport : PMIOPort  Orientation=left  Port=1  Side=Right
  wires:
  SIZED_INPUT_PORT/1 -> MSB_SIGNAL_BLOCK/1
  Ground/1 -> actuator/1
  connections:
  actuator/RConn1 -- pmioport/RConn1

== system mblibv1/Sensors &  Actuators/Joint Initial Condition ==
  Ground : Ground
  actuator : Actuator  PhysicalDomain=generic  SubClassName=Unknown  PortType=Generic
  pmioport : PMIOPort  Orientation=left  Port=1  Side=Right
  wires:
  Ground/1 -> actuator/1
  connections:
  actuator/RConn1 -- pmioport/RConn1

== system mblibv1/Sensors &  Actuators/Joint Sensor ==
  MSB_SIGNAL_BLOCK : Constant  Value=0
  Terminator : Terminator
  sensor : Sensor  Tag=Factory sensor  PhysicalDomain=generic  SubClassName=Unknown  PortType=Generic
  pmioport : PMIOPort  Port=1  Side=Left
  Out1 : Outport
  wires:
  sensor/1 -> Terminator/1
  MSB_SIGNAL_BLOCK/1 -> Out1/1
  connections:
  pmioport/RConn1 -- sensor/LConn1

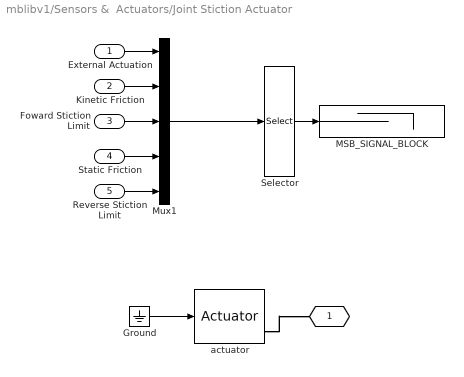
== system mblibv1/Sensors &  Actuators/Joint Stiction Actuator ==
  External Actuation : Inport  Port=1  PortDimensions=1  LatchInput=off
  Kinetic Friction : Inport  Port=2  PortDimensions=1  LatchInput=off
  Foward Stiction Limit : Inport  Port=3  PortDimensions=1  LatchInput=off
  Static Friction : Inport  Port=4  PortDimensions=1  LatchInput=off
  Reverse Stiction Limit : Inport  Port=5  PortDimensions=1  LatchInput=off
  Ground : Ground
  MSB_SIGNAL_BLOCK : Terminator
  Mux1 : Mux  Inputs=5
  Selector : Selector  Elements=[1 2 4 5 3]  InputPortWidth=5
  actuator : Actuator  PhysicalDomain=generic  SubClassName=Unknown  PortType=Generic
  " " : PMIOPort  Orientation=left  Port=1  Side=Right
  wires:
  Mux1/1 -> Selector/1
  Reverse Stiction Limit/1 -> Mux1/5
  Static Friction/1 -> Mux1/4
  Foward Stiction Limit/1 -> Mux1/3
  Kinetic Friction/1 -> Mux1/2
  External Actuation/1 -> Mux1/1
  Ground/1 -> actuator/1
  Selector/1 -> MSB_SIGNAL_BLOCK/1
  connections:
  actuator/RConn1 -- " "/RConn1

== system mblibv1/Sensors &  Actuators/Variable Mass & Inertia Actuator ==
  SIZED_INPUT_PORT : Inport  Port=1  PortDimensions=1  LatchInput=off
  Ground : Ground
  MSB_SIGNAL_BLOCK : Terminator
  actuator : Actuator  PhysicalDomain=generic  SubClassName=Unknown  PortType=Generic
  pmioport : PMIOPort  Orientation=left  Port=1  Side=Right
  wires:
  SIZED_INPUT_PORT/1 -> MSB_SIGNAL_BLOCK/1
  Ground/1 -> actuator/1
  connections:
  actuator/RConn1 -- pmioport/RConn1

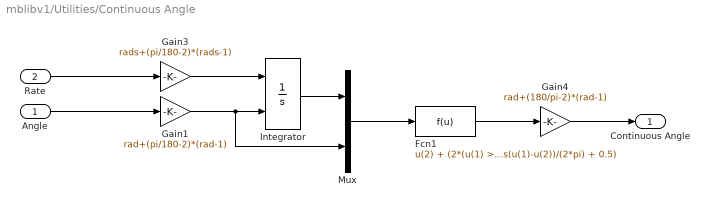
== system mblibv1/Utilities/Continuous Angle ==
  Angle : Inport  Port=1  LatchInput=off
  Rate : Inport  Port=2  LatchInput=off
  Fcn1 : Fcn  Expr=u(2) + (2*(u(1) > u(2)) - 1)*2*pi*floor(abs(u(1)-u(2))/(2*pi) + 0.5)
  Gain1 : Gain  Gain=rad+(pi/180-2)*(rad-1)  SaturateOnIntegerOverflow=on
  Gain3 : Gain  Gain=rads+(pi/180-2)*(rads-1)  SaturateOnIntegerOverflow=on
  Gain4 : Gain  Gain=rad+(180/pi-2)*(rad-1)  SaturateOnIntegerOverflow=on
  Integrator : Integrator  InitialConditionSource=external  AbsoluteTolerance=1e-3  ZeroCross=off
  Mux : Mux  Inputs=2
  Continuous Angle : Outport
  wires:
  Gain4/1 -> Continuous Angle/1
  Gain3/1 -> Integrator/1
  Integrator/1 -> Mux/1
  Mux/1 -> Fcn1/1
  Fcn1/1 -> Gain4/1
  Rate/1 -> Gain3/1
  Angle/1 -> Gain1/1
  Gain1/1 -> Integrator/2, Mux/2

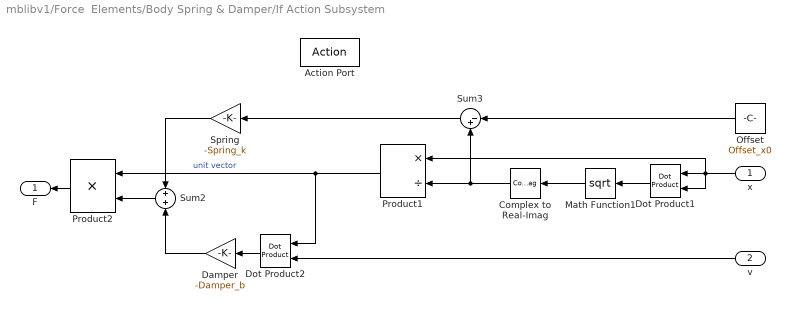
== system mblibv1/Force  Elements/Body Spring & Damper/If Action Subsystem ==
  x : Inport  Orientation=left  Port=1  LatchInput=off
  v : Inport  Orientation=left  Port=2  LatchInput=off
  Action Port : ActionPort
  Complex to Real-Imag : ComplexToRealImag  Orientation=left  Output=Real
  Damper : Gain  Orientation=left  Gain=-Damper_b  SaturateOnIntegerOverflow=on
  Dot Product1 : simulink/Math Operations/Dot Product  Orientation=left  OutDataType=sfix(16)  OutScaling=2^-10  DoSatur=off
  Dot Product2 : simulink/Math Operations/Dot Product  Orientation=left  OutDataType=sfix(16)  OutScaling=2^-10  DoSatur=off
  Math Function1 : Math  Orientation=left  Operator=sqrt  OutputSignalType=complex  SaturateOnIntegerOverflow=on
  Offset : Constant  Orientation=left  Value=Offset_x0  VectorParams1D=off
  Product1 : Product  Orientation=left  Inputs=*/  SaturateOnIntegerOverflow=on
  Product2 : Product  Orientation=left  SaturateOnIntegerOverflow=on
  Spring : Gain  Orientation=left  Gain=-Spring_k  SaturateOnIntegerOverflow=on
  Sum2 : Sum  Orientation=left  SaturateOnIntegerOverflow=on
  Sum3 : Sum  Orientation=left  Inputs=|-+  SaturateOnIntegerOverflow=on
  F : Outport  Orientation=left
  wires:
  Complex to Real-Imag/1 -> Sum3/2, Product1/2
  Math Function1/1 -> Complex to Real-Imag/1
  Offset/1 -> Sum3/1
  Spring/1 -> Sum2/1
  Sum2/1 -> Product2/2
  Damper/1 -> Sum2/2
  Dot Product2/1 -> Damper/1
  v/1 -> Dot Product2/2
  Product1/1 -> Dot Product2/1, Product2/1  "unit vector"
  Sum3/1 -> Spring/1
  Dot Product1/1 -> Math Function1/1
  x/1 -> Dot Product1/1, Dot Product1/2, Product1/1
  Product2/1 -> F/1

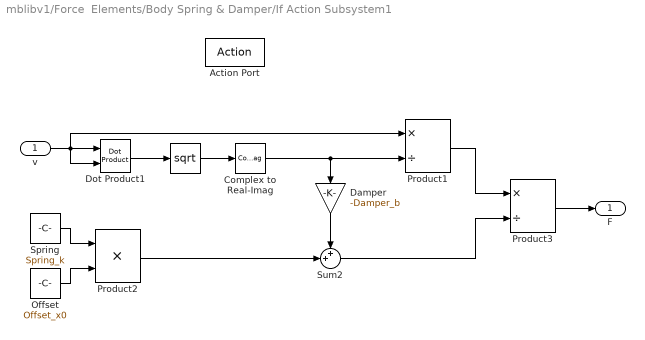
== system mblibv1/Force  Elements/Body Spring & Damper/If Action Subsystem1 ==
  v : Inport  Port=1  LatchInput=off
  Action Port : ActionPort
  " " : Math  Operator=sqrt  OutputSignalType=complex  SaturateOnIntegerOverflow=on
  Complex to Real-Imag : ComplexToRealImag  Output=Real
  Damper : Gain  Orientation=down  Gain=-Damper_b  SaturateOnIntegerOverflow=on
  Dot Product1 : simulink/Math Operations/Dot Product  OutDataType=sfix(16)  OutScaling=2^-10  DoSatur=off
  Offset : Constant  Value=Offset_x0  VectorParams1D=off
  Product1 : Product  Inputs=*/  SaturateOnIntegerOverflow=on
  Product2 : Product  SaturateOnIntegerOverflow=on
  Product3 : Product  Inputs=*/  SaturateOnIntegerOverflow=on
  Spring : Constant  Value=Spring_k  VectorParams1D=off
  Sum2 : Sum  Inputs=++|  SaturateOnIntegerOverflow=on
  F : Outport
  wires:
  Complex to Real-Imag/1 -> Damper/1, Product1/2
  " "/1 -> Complex to Real-Imag/1
  v/1 -> Dot Product1/1, Dot Product1/2, Product1/1
  Product1/1 -> Product3/1
  Damper/1 -> Sum2/1
  Spring/1 -> Product2/1
  Offset/1 -> Product2/2
  Product2/1 -> Sum2/2
  Dot Product1/1 -> " "/1
  Sum2/1 -> Product3/2
  Product3/1 -> F/1

== system mblibv1/Force  Elements/Body Spring & Damper/If Action Subsystem2 ==
  Action Port : ActionPort
  Assertion : Assertion  AssertionFailFcn=errordlg('Singularity in Body Spring & Damper: Zero relative displacement and velocity, but nonzero natural length. Force has no defined direction. Separate the two coordinate systems at each end of the spring so the spring has nonzero initial length.','Singularity in Body Spring & Damper');  StopWhenAssertionFail=off
  Constant : Constant
  Offset : Constant  Value=0  VectorParams1D=off
  Stop Simulation : Stop
  wires:
  Constant/1 -> Stop Simulation/1
  Offset/1 -> Assertion/1

== system mblibv1/Force  Elements/Body Spring & Damper/If Action Subsystem4 ==
  Action Port : ActionPort
  " " : Constant  Value=[0 0 0]  VectorParams1D=off
  Out1 : Outport  InitialOutput=[0 0 0]
  wires:
  " "/1 -> Out1/1
